simulink model "Preprocessing"  (R2022a)
settings: Solver=VariableStepAuto  StartTime=0.0  StopTime=10.0  RelTol=1e-3
model workspace (MAT data in the model file):
  K = [2.51632988536 0.393907730554 2.24903461301 0.177004257907 -4.17656095855]
  LateralControllers_FeedbackGainLQR = Simulink.Parameter
  LateralControllers_FeedbackGainLQR.Value = [2.51632988536 0.393907730554 2.24903461301 0.177004257907]
  LateralControllers_FeedbackGainLQR.Description = 'LQR feedback gain [K_e1, K_de1, K_e2, K_de2, K_int]'
  LateralControllers_FeedbackGainLQR.DataType = 'double'
  LateralControllers_FeedbackGainLQR.Complexity = 'real'
  LateralControllers_FeedbackGainLQR.Dimensions = [1 4]
  car.m = 1465
  car.Iz = 1600
  car.lf = 1.85
  car.lr = 2.43
  car.Caf = 80000
  car.Car = 80000
undefined symbols (not defined in the file): Vehicle_SteeringGearRatio
settings Model: Creator=krisz  LastModifiedBy=krisz

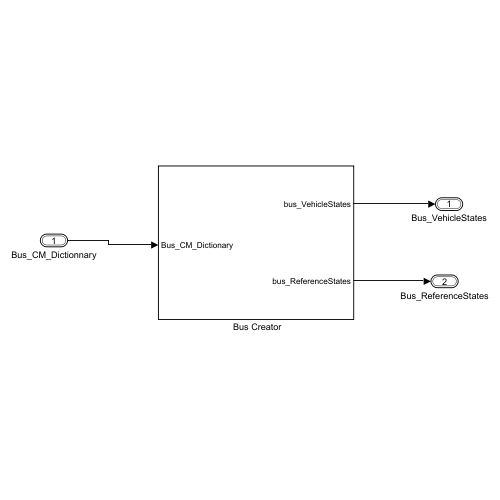
[thumbnail: Simulink's stored preview of the top-level diagram]
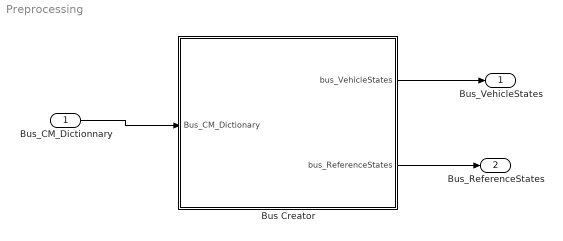
== system Preprocessing ==
  Bus_CM_Dictionnary : Inport  OutDataTypeStr=Bus: Bus_CM_Dictionary
  " Bus Creator" : Subsystem
  Bus_VehicleStates : Outport  OutDataTypeStr=Bus: bus_VehicleStates
  Bus_ReferenceStates : Outport  Port=2  OutDataTypeStr=Bus: bus_ReferenceStates
  wires:
  Bus_CM_Dictionnary/1 -> " Bus Creator"/1(Bus_CM_Dictionary)
  " Bus Creator"/1(bus_VehicleStates) -> Bus_VehicleStates/1
  " Bus Creator"/2(bus_ReferenceStates) -> Bus_ReferenceStates/1

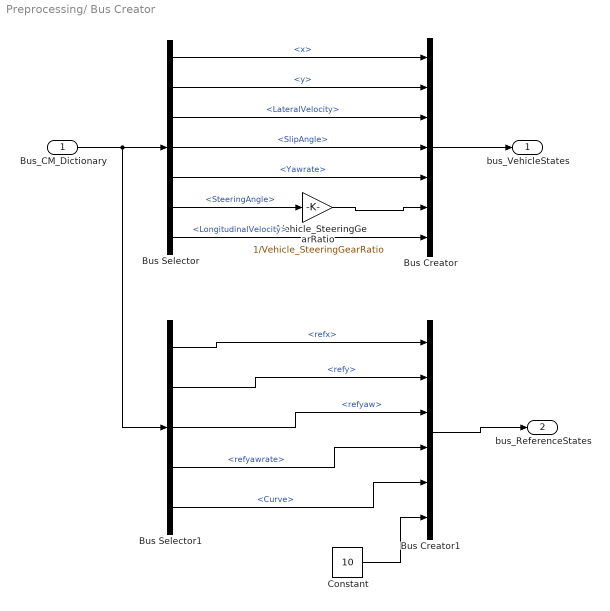
== system Preprocessing/ Bus Creator ==
  Bus_CM_Dictionary : Inport  OutDataTypeStr=Bus: Bus_CM_Dictionary
  1/Vehicle_SteeringGearRatio : Gain  Gain=1/Vehicle_SteeringGearRatio
  Bus Creator : BusCreator  Inputs=7
  Bus Creator1 : BusCreator  Inputs=6
  Bus Selector : BusSelector  OutputSignals=x,y,LateralVelocity,SlipAngle,Yawrate,SteeringAngle,LongitudinalVelocity
  Bus Selector1 : BusSelector  OutputSignals=refx,refy,refyaw,refyawrate,Curve
  Constant : Constant  Value=10
  bus_VehicleStates : Outport  OutDataTypeStr=Bus: bus_VehicleStates
  bus_ReferenceStates : Outport  Port=2  OutDataTypeStr=Bus: bus_ReferenceStates
  wires:
  Bus Creator/1 -> bus_VehicleStates/1
  Bus_CM_Dictionary/1 -> Bus Selector1/1, Bus Selector/1
  Bus Selector/1 -> Bus Creator/1  "<x>"
  Bus Selector/3 -> Bus Creator/3  "<LateralVelocity>"
  Bus Selector/4 -> Bus Creator/4  "<SlipAngle>"
  Bus Selector/5 -> Bus Creator/5  "<Yawrate>"
  1/Vehicle_SteeringGearRatio/1 -> Bus Creator/6
  Bus Selector/6 -> 1/Vehicle_SteeringGearRatio/1  "<SteeringAngle>"
  Bus Selector/7 -> Bus Creator/7  "<LongitudinalVelocity>"
  Bus Selector/2 -> Bus Creator/2  "<y>"
  Bus Creator1/1 -> bus_ReferenceStates/1
  Bus Selector1/1 -> Bus Creator1/1  "<refx>"
  Bus Selector1/2 -> Bus Creator1/2  "<refy>"
  Bus Selector1/3 -> Bus Creator1/3  "<refyaw>"
  Bus Selector1/4 -> Bus Creator1/4  "<refyawrate>"
  Bus Selector1/5 -> Bus Creator1/5  "<Curve>"
  Constant/1 -> Bus Creator1/6
